simulink model "test02_sensor_bis"  (R2013b)
settings: Solver=FixedStepDiscrete  StartTime=0.0  StopTime=10.0  FixedStep=0.05  RelTol=1e-3
InitFcn:
  | load 'variabili.mat'
  | 
  | %eseguo il punto m per inizializzare la porta di imput
  | %senza load, loas solo con .mat
  | variabili_porta_imput
StopFcn:
  | tempo = yout.time;
  | 
  | uscita = yout.signals.values;
  | 
  | plot(tempo,uscita)
values from neighbouring files (symbols this model uses):
  var = [0,45,90]    [variabili.m]    (also in variabili.mat = [0 45 90])
  var2 = [0.5,3.6,4.5]    [variabili.m]    (also in variabili.mat = [0.5 3.6 4.5])
settings Model: Creator=training-it  LastModifiedBy=training-it
settings DataIOCC: LoadExternalInput=on  SaveFormat=StructureWithTime

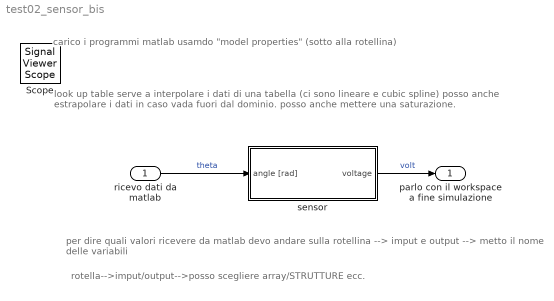
== system test02_sensor_bis ==
  note: rotella-->imput/output-->posso scegliere array/STRUTTURE ecc.
  note: per dire quali valori ricevere da matlab devo andare sulla rotellina --> imput e output --> metto il nome delle variabili
  note: look up table serve a interpolare i dati di una tabella (ci sono lineare e cubic spline)
      | posso anche estrapolare i dati in caso vada fuori dal dominio. posso anche mettere una saturazione.
  note: carico i programmi matlab usamdo "model properties" (sotto alla rotellina)
  ricevo dati da matlab : Inport
  sensor : Subsystem
  parlo con il workspace a fine simulazione : Outport
  Scope : SignalViewerScope  IOType=viewer  NumInputPorts=2  RefreshTime=0.035000
      settings: YMin=-5~-5  YMax=5~5
  wires:
  sensor/1(voltage) -> parlo con il workspace a fine simulazione/1  "volt"
  ricevo dati da matlab/1 -> sensor/1(angle [rad])  "theta"

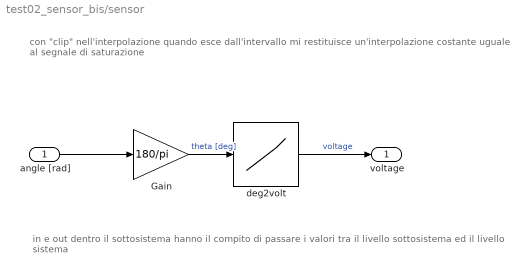
== system test02_sensor_bis/sensor ==
  note: in e out dentro il sottosistema hanno il compito di passare i valori tra il livello sottosistema ed il livello sistema
  note: con "clip" nell'interpolazione quando esce dall'intervallo mi restituisce un'interpolazione costante uguale al segnale di saturazione
  angle [rad] : Inport
  Gain : Gain  Gain=180/pi
  deg2volt : Lookup_n-D  NumberOfTableDimensions=1  BreakpointsForDimension1=var  Table=var2  TableMin=[0.5]  TableMax=[4.5]  ExtrapMethod=Clip  InternalRulePriority=Speed  RndMeth=Simplest  InputSameDT=on
  voltage : Outport
  wires:
  angle [rad]/1 -> Gain/1
  Gain/1 -> deg2volt/1  "theta [deg]"
  deg2volt/1 -> voltage/1  "voltage"
